simulink model "H2DFRL_LExCI_env"  (R2023a)
settings: Solver=FixedStepAuto  StartTime=0.0  StopTime=50  FixedStep=0.08  RelTol=1e-3
values from neighbouring files (symbols this model uses):
  action_mean_selector_ppo = 1:num_actions    [ReinforcementLearningBlockInit_H2DFRL.m]
  action_sampling_mode = 1    [ReinforcementLearningBlockInit_H2DFRL.m]
  action_selector_ddpg = 1:num_actions    [ReinforcementLearningBlockInit_H2DFRL.m]
  action_std_selector_ppo = 1:num_actions    [ReinforcementLearningBlockInit_H2DFRL.m]
  action_type = 1    [ReinforcementLearningBlockInit_H2DFRL.m]
  C2C_NMPC = init_C2C_NMPC_H2DF(C2C_NMPC.expdata)    [init_H2DFRL_GRU.m]
  LowerLimit = ([0.17e-3;350;-1;1.5e-3] - C2C_NMPC.Normalization.controls.mean)./(C2C_NMPC.Normalization.controls.std)    [init_H2DFRL_GRU.m]
  num_actions = 4    [ReinforcementLearningBlockInit_H2DFRL.m]
  rl_algorithm = 2    [ReinforcementLearningBlockInit_H2DFRL.m]
  Ts = 0.08    [init_H2DFRL_GRU.m]
  UpperLimit = ([0.5e-3;900;0;5.5e-3] - C2C_NMPC.Normalization.controls.mean)./(C2C_NMPC.Normalization.controls.std)    [init_H2DFRL_GRU.m]
undefined symbols (not defined in the file or in its folder): CA50_offset, DiscIntNeverNeededParam, enable_CA50_noise, enable_CA50_offset, enable_IMEP_noise, enable_IMEP_offset, IMEP_offset, NUMBER_OF_ACTIONS
libraries: simulink x15, dspsrcs4 x4, slctrlblks x2, statsLibrary x1
(part 2 of 4)

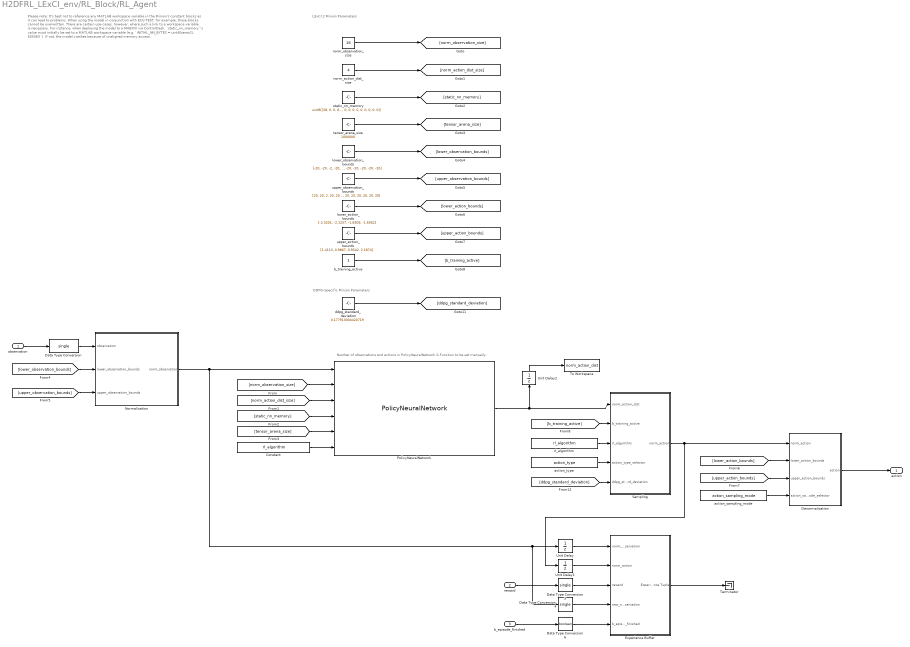
== system H2DFRL_LExCI_env/RL_Block/RL_Agent ==
  note: LExCI 2 Minion Parameters
  note: DDPG-Specific Minion Parameters
  note: Number of observations and actions in PolicyNeuralNetwork S-Function to be set manually.
  note: Please note:
      |
      | It's best not to reference any MATLAB workspace variable in the Minion's constant blocks as it can lead to
      | problems. When using the model in conjunction with ECU-TEST, for example, those blocks cannot be
      | overwritten.
      |
      | There are certain use-cases, however, where such a link to a workspace variable is necessary. For
      | instance, when deploying the model to a MABXIII via ControlDesk, `static_nn_memory`'s value must
      | initially be set to a MATLAB workspace variable (e.g. `INITIAL_NN_BYTES = uint8(zeros(1, 65536))`). If
      | not, the model crashes because of unaligned memory access.
  observation : Inport
  reward : Inport  Port=2
  b_episode_finished : Inport  Port=3
  Constant : Constant  Value=rl_algorithm  OutDataTypeStr=uint32
  Data Type Conversion : DataTypeConversion  OutDataTypeStr=single  SaturateOnIntegerOverflow=off  RndMeth=Floor
  Data Type Conversion3 : DataTypeConversion  OutDataTypeStr=single  SaturateOnIntegerOverflow=off  RndMeth=Floor
  Data Type Conversion4 : DataTypeConversion  OutDataTypeStr=single  SaturateOnIntegerOverflow=off  RndMeth=Floor
  Data Type Conversion6 : DataTypeConversion  OutDataTypeStr=boolean  SaturateOnIntegerOverflow=off  RndMeth=Floor
  Denormalization : Subsystem
  Experience Buffer : Subsystem
  Normalization : Subsystem
  PolicyNeuralNetwork : S-Function  InitFcn=try, set_param(gcb,'FunctionName','PolicyNeuralNetwork'), end  FunctionName=PolicyNeuralNetwork  SFunctionModules=PolicyNeuralNetwork_wrapper.cpp activations activations_common add add_common add_n arg_min_max assign_variable batch_to_space_nd broadcast_args broadcast_to call_once cast ceil circular_buffer circular_buffer_common comparisons concatenation conv conv_common cumsum depth_to_space depthwise_conv depthwise_conv_common dequantize dequantize_common detection_postprocess div elementwise elu ethosu exp expand_dims fill floor floor_div floor_mod fully_connected fully_connected_common gather gather_nd hard_swish hard_swish_common if kernel_runner kernel_util_micro l2norm l2_pool_2d leaky_relu leaky_relu_common logical logical_common logistic logistic_common log_softmax lstm_eval maximum_minimum micro_tensor_utils mirror_pad mul mul_common neg pack pad pooling pooling_common prelu prelu_common quantize quantize_common read_variable reduce reduce_common reshape resize_bilinear resize_nearest_neighbor round shape slice softmax softmax_common space_to_batch_nd space_to_depth split split_v squared_difference squeeze strided_slice sub sub_common svdf svdf_common tanh transpose transpose_conv unidirectional_sequence_lstm unpack var_handle while zeros_like flatbuffer_conversions op_resolver tensor_utils error_reporter schema_utils kernel_util portable_tensor_utils quantization_util common memory_helpers all_ops_resolver micro_graph micro_error_reporter micro_context micro_profiler test_helpers recording_micro_allocator micro_interpreter micro_time micro_resource_variable test_helper_custom_ops flatbuffer_utils mock_micro_graph debug_log micro_allocation_info system_setup micro_allocator micro_string micro_utils fake_micro_context persistent_arena_buffer_allocator recording_single_arena_buffer_allocator non_persistent_arena_buffer_allocator single_arena_buffer_allocator greedy_memory_planner linear_memory_planner non_persistent_buffer_planner_shim  SFunctionDeploymentMode=off  EnableBusSupport=off  mask(S-Function Builder){}
      mask help: Simulink:masks:SFunctionBuilder_MD
      mask init:
      | val = [[.9  0.75 0.75 1 1 .9 .9 1]',[1 1 0.75 0.75 .9 .9 1 .9]'];try , sys = get_param(gcb,'SfunBuilderFcnName');if isempty(sys), sys = get_param(gcb,'FunctionName'); end,catch, sys = get_param(gcb,'FunctionName'); end
      settings: CopyFcn=set_param(gcbh,'LinkStatus','none')  PreSaveFcn=try, set_param(gcb,'FunctionName','PolicyNeuralNetwork'), end  OpenFcn=sfunctionwizard(gcbh)
      mask Display: plot(val(:,1),val(:,2)),disp(sys),port_label('input',1,'norm_observation'),port_label('input',2,'norm_observation_size'),port_label('input',3,'norm_action_dist_size'),port_label('input',4,'static_nn_memory'),port_label('input',5,'tensor_arena_size'),port_label('input',6,'rl_algorithm'),port_label('output',1,'norm_action_dist')
  Sampling : Subsystem
  Terminator : Terminator
  To Workspace : ToWorkspace  VariableName=norm_action_dist  SampleTime=-1
  Unit Delay : UnitDelay  InitialCondition=-1*ones(16,1)  SampleTime=-1  HasFrameUpgradeWarning=on
  Unit Delay1 : UnitDelay  InitialCondition=-1*ones(4,1)  SampleTime=-1  HasFrameUpgradeWarning=on
  Unit Delay2 : UnitDelay  InitialCondition=-1*ones(4,1)  SampleTime=-1  HasFrameUpgradeWarning=on
  action_sampling_mode : Constant  Value=action_sampling_mode  OutDataTypeStr=uint8
  action_type : Constant  Value=action_type  OutDataTypeStr=uint8
  b_training_active : Constant  OutDataTypeStr=boolean
  ddpg_standard_deviation : Constant  Value=0.177913004420719  OutDataTypeStr=single
  lower_action_bounds : Constant  Value=[-2.3201, -2.1257, -1.8309, -1.6562]  OutDataTypeStr=single
  lower_observation_bounds : Constant  Value=[-20, -20, -2, -20, -20, -20, -2, -20, -20, -20, -20, -20, -20, -20, -20, -20]  OutDataTypeStr=single
  norm_action_dist_size : Constant  Value=4  OutDataTypeStr=uint32
  norm_observation_size : Constant  Value=16  OutDataTypeStr=uint32
  rl_algorithm : Constant  Value=rl_algorithm  OutDataTypeStr=uint8
  static_nn_memory : Constant  Value=uint8([28, 0, 0, 0, 84, 70, 76, 51, 0, 0, 18, 0, 28, 0, 24, 0, 20, 0, 16, 0, 12, 0, 8, 0, 0, 0, 4, 0, 18, 0, 0, 0, 24, 0, 0, 0, 104, 0, 0, 0, 140, 87, 0, 0, 156, 87, 0, 0, 228, 91, 0, 0, 3, 0, 0, 0, 2, 0, 0, 0, 44, 0, 0, 0, 4, 0, 0, 0, 40, 167, 255, 255, 12, 0, 0, 0, 4, 0, 0, 0, 19, 0, 0, 0, 67, 79, 78, 86, 69, 82, 83, 73, 79, 78, 95, 77, 69, 84, 65, 68, 65, 84, 65, 0, 76, 167, 255, 255, 11, 0, 0, 0, 4, 0, 0, 0, 19, 0, 0, 0, 109, 105, 110, 95, 114, 117, 110, 116, 105, 109, 101, 95, 118, 101, 114, 115, 105, 111, 110, 0, 13, 0, 0, 0, 32, 87, 0, 0, 0, 87, 0, 0, 232, 82, 0, 0, 216, 81, 0, 0, 200, 17, 0, 0, 184, 16, 0, 0, 168, 0, 0, 0, 160, 0, 0, 0, 152, 0, 0, 0, 144, 0, 0, 0, 136, 0, 0, 0, 104, 0, 0, 0, 4, 0, 0, 0, 54, 169, 255, 255, 4, 0, 0, 0, 84, 0, 0, 0, 12, 0, 0, 0, 8, 0, 14, 0, 8, 0, 4, 0, 8, 0, 0, 0, 16, 0, 0, 0, 36, 0, 0, 0, 0, 0, 6, 0, 8, 0, 4, 0, 6, 0, 0, 0, 4, 0, 0, 0, 0, 0, 0, 0, 0, 0, 10, 0, 16, 0, 12, 0, 8, 0, 4, 0, 10, 0, 0, 0, 2, 0, 0, 0, 2, 0, 0, 0, 4, 0, 0, 0, 6, 0, 0, 0, 50, 46, 49, 49, 46, 48, 0, 0, 150, 169, 255, 255, 4, 0, 0, 0, 16, 0, 0, 0, 49, 46, 53, 46, 48, 0, 0, 0, 0, 0, 0, 0, 0, 0, 0, 0, 80, 165, 255, 255, 84, 165, 255, 255, 88, 165, 255, 255, 92, 165, 255, 255, 194, 169, 255, 255, 4, 0, 0, 0, 0, 16, 0, 0, 161, 135, 150, 61, 207, 91, 94, 62, 33, 223, 11, 61, 131, 146, 51, 188, 56, 213, 137, 61, 52, 31, 98, 62, 248, 70, 89, 189, 67, 75, 100, 190, 48, 127, 73, 190, 134, 205, 105, 59, 50, 123, 133, 61, 199, 172, 162, 59, 194, 235, 91, 190, 189, 20, 50, 61, 106, 38, 17, 190, 126, 161, 200, 189, 83, 157, 96, 189, 119, 253, 3, 60, 237, 225, 238, 188, 244, 226, 153, 190, 140, 17, 59, 190, 70, 145, 98, 189, 71, 208, 20, 190, 70, 171, 72, 190, 194, 82, 25, 190, 155, 130, 79, 190, 205, 234, 129, 189, 74, 210, 190, 61, 77, 151, 253, 61, 18, 180, 205, 61, 237, 153, 251, 61, 11, 110, 224, 187, 145, 76, 13, 62, 131, 216, 156, 188, 250, 7, 45, 62, 2, 3, 156, 190, 129, 0, 173, 62, 156, 169, 48, 190, 10, 214, 94, 62, 97, 61, 181, 62, 79, 156, 252, 188, 129, 162, 120, 190, 230, 34, 47, 62, 121, 152, 69, 62, 254, 215, 46, 62, 117, 140, 35, 190, 29, 11, 141, 61, 13, 123, 141, 189, 228, 98, 5, 62, 112, 233, 6, 61, 25, 136, 5, 190, 51, 49, 207, 59, 126, 102, 241, 61, 148, 149, 157, 189, 200, 67, 246, 189, 178, 140, 185, 62, 178, 124, 133, 62, 227, 198, 134, 190, 123, 249, 13, 189, 237, 126, 131, 62, 10, 17, 213, 61, 54, 120, 174, 61, 81, 191, 222, 60, 216, 115, 22, 62, 69, 179, 144, 190, 87, 153, 106, 61, 220, 120, 6, 188, 15, 68, 194, 189, 170, 91, 78, 62, 233, 241, 148, 62, 218, 55, 143, 62, 1, 240, 76, 62, 159, 95, 171, 61, 11, 128, 192, 60, 211, 193, 3, 62, 220, 174, 74, 62, 202, 36, 186, 189, 252, 231, 237, 61, 251, 167, 187, 61, 104, 116, 213, 60, 97, 31, 148, 190, 163, 31, 181, 190, 121, 16, 14, 62, 30, 99, 71, 189, 180, 101, 38, 189, 200, 172, 49, 190, 24, 246, 139, 190, 237, 45, 186, 62, 208, 108, 29, 189, 247, 203, 15, 190, 132, 35, 16, 190, 146, 226, 125, 62, 253, 7, 61, 62, 110, 146, 1, 62, 43, 208, 74, 61, 49, 163, 43, 190, 18, 8, 102, 61, 7, 4, 105, 190, 213, 164, 136, 190, 29, 115, 126, 190, 231, 25, 238, 61, 107, 120, 116, 190, 81, 18, 143, 62, 0, 139, 65, 190, 56, 134, 131, 189, 116, 53, 150, 189, 24, 102, 14, 190, 176, 98, 107, 62, 84, 192, 73, 62, 78, 102, 80, 62, 147, 89, 219, 188, 167, 106, 56, 62, 67, 28, 234, 188, 120, 159, 50, 62, 137, 217, 22, 190, 133, 249, 10, 61, 184, 70, 79, 187, 226, 72, 124, 189, 107, 111, 227, 61, 232, 132, 151, 60, 147, 42, 222, 61, 14, 188, 187, 61, 103, 13, 197, 189, 156, 242, 249, 61, 24, 29, 19, 61, 54, 221, 197, 60, 190, 220, 30, 62, 35, 52, 15, 190, 130, 57, 209, 190, 165, 29, 137, 59, 68, 230, 151, 189, 162, 248, 40, 190, 208, 137, 231, 189, 158, 148, 170, 186, 184, 152, 185, 60, 75, 35, 84, 62, 27, 167, 130, 60, 82, 125, 77, 190, 24, 186, 222, 61, 164, 246, 140, 189, 240, 212, 97, 190, 255, 235, 232, 189, 202, 109, 57, 62, 6, 83, 68, 62, 116, 97, 194, 61, 19, 79, 63, 61, 242, 151, 195, 189, 95, 105, 16, 190, 141, 97, 189, 61, 128, 152, 162, 62, 249, 61, 78, 190, 89, 71, 4, ...(+227019 chars)])  OutDataTypeStr=uint8
  tensor_arena_size : Constant  Value=1000000  OutDataTypeStr=uint32
  upper_action_bounds : Constant  Value=[1.4113, 0.9867, 0.9542, 2.1874]  OutDataTypeStr=single
  upper_observation_bounds : Constant  Value=[20, 20, 2, 20, 20, 20, 2, 20, 20, 20, 20, 20, 20, 20, 20, 20]  OutDataTypeStr=single
  action : Outport
  wires:
  upper_action_bounds/1 -> [upper_action_bounds]
  PolicyNeuralNetwork/1 -> Unit Delay2/1, Sampling/1(norm_action_dist)
  upper_observation_bounds/1 -> [upper_observation_bounds]
  lower_action_bounds/1 -> [lower_action_bounds]
  [upper_observation_bounds] -> Normalization/3(upper_observation_bounds)
  [tensor_arena_size] -> PolicyNeuralNetwork/5
  b_episode_finished/1 -> Data Type Conversion6/1
  Unit Delay/1 -> Experience Buffer/1(norm_observation)
  [norm_observation_size] -> PolicyNeuralNetwork/2
  Data Type Conversion6/1 -> Experience Buffer/5(b_episode_finished)
  Unit Delay1/1 -> Experience Buffer/2(norm_action)
  Data Type Conversion3/1 -> Experience Buffer/3(reward)
  norm_observation_size/1 -> [norm_observation_size]
  Data Type Conversion/1 -> Normalization/1(observation)
  lower_observation_bounds/1 -> [lower_observation_bounds]
  Data Type Conversion4/1 -> Experience Buffer/4(new_norm_observation)
  reward/1 -> Data Type Conversion3/1
  norm_action_dist_size/1 -> [norm_action_dist_size]
  static_nn_memory/1 -> [static_nn_memory]
  Normalization/1(norm_observation) -> Unit Delay/1, Data Type Conversion4/1, PolicyNeuralNetwork/1
  observation/1 -> Data Type Conversion/1
  [norm_action_dist_size] -> PolicyNeuralNetwork/3
  [lower_observation_bounds] -> Normalization/2(lower_observation_bounds)
  tensor_arena_size/1 -> [tensor_arena_size]
  Experience Buffer/1(Experience Tuple) -> Terminator/1
  Sampling/1(norm_action) -> Unit Delay1/1, Denormalization/1(norm_action)
  Denormalization/1(action) -> action/1
  [lower_action_bounds] -> Denormalization/2(lower_action_bounds)
  [upper_action_bounds] -> Denormalization/3(upper_action_bounds)
  [static_nn_memory] -> PolicyNeuralNetwork/4
  b_training_active/1 -> [b_training_active]
  [b_training_active] -> Sampling/2(b_training_active)
  ddpg_standard_deviation/1 -> [ddpg_standard_deviation]
  action_sampling_mode/1 -> Denormalization/4(action_sampling_mode_selector)
  action_type/1 -> Sampling/4(action_type_selector)
  rl_algorithm/1 -> Sampling/3(rl_algorithm)
  [ddpg_standard_deviation] -> Sampling/5(ddpg_standard_deviation)
  Constant/1 -> PolicyNeuralNetwork/6
  Unit Delay2/1 -> To Workspace/1
